simulink library "powerlib_models"  (Simulink 6.0)
settings: Solver=ode45  SolverMode=SingleTasking  StartTime=0.0  StopTime=10.0  RelTol=1e-3
values from neighbouring files (symbols this model uses):
  Ts = get(handles.edit1,'string')    [powergui.m]
undefined symbols (not defined in the file or in its folder): A, a0, a1, a2, a3, a4, a5, Ac, Amplitude, Amplitudes, B, BaseCurrent, BaseFlux, Bc, C, Capacitance, Cc, Columns, ConnectionType, Cs, ctrl, current, Current, damp, Dc, Dd, DiscIntNeverNeededParam, dref, dwo, exc, excAxis, F, Flux, fnom, Frequency, FreqVps, Gain1, gate, GH, GHd, GI, GId, GL, GLd, H, HarmonicGeneration, HT, hyd, I1_init, ib, ib2, Id1o, Inductance, InitialFlux, InitialSlope, io, Iq1o, isfinite, j, J ... (+138)
libraries: powerlib_models x32, powerlib_extras x4
(part 1 of 11)
settings Model: RequirementInfo=9  Creator=Patrice Brunelle  LastModifiedBy=batserve  ModifiedComment=-- Tue Aug 22 15:28:00 2000 -- Version 1.317  ModifiedHistory=Powerlib_models  ExtModeAutoUpdateStatusClock=off
settings OptimizationCC: BooleanDataType=off
settings DebuggingCC: SolverPrmCheckMsg=none
settings HardwareCC: TargetUnknown=on

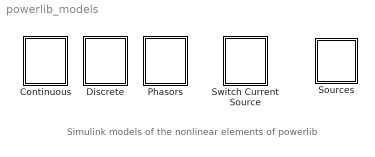
== system powerlib_models ==
  note: Simulink models of the nonlinear elements of powerlib
  Continuous : Subsystem
  Discrete : Subsystem
  Phasors : Subsystem
  Sources : Subsystem
  Switch Current Source : Subsystem

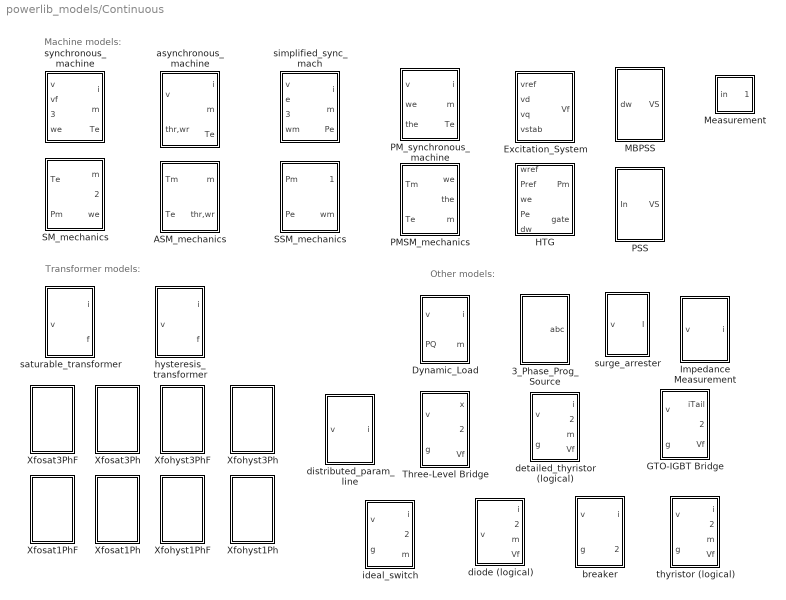
== system powerlib_models/Continuous ==
  note: Machine models:
  note: Transformer models:
  note: Other models:
  3_Phase_Prog_Source : Subsystem
  ASM_mechanics : Subsystem
  Dynamic_Load : Subsystem
  Excitation_System : Subsystem  mask(Excitation System){tr=tr, reg=reg, exc=exc, tgr=tgr, damp=damp, sat=sat, lim=lim, v0=v0}
      mask prompts: tr "Low-pass filter time constant Tr(s):"; reg "Regulator gain and time constant [ Ka()  Ta(s) ]:"; exc "Exciter  [ Ke()  Te(s) ]:"; tgr "Transient gain reduction [ Tb(s)  Tc(s) ]:"; damp "Damping filter gain and time constant  [ Kf()  Tf(s)  ]:"; sat "Field saturation parameters [ A, B ]:"; lim "Regulator output limits and gain [ Efmin, Efmax (p.u.), Kp() ]:"; v0 "Initial values of terminal voltage  and field voltage [ Vt0 (pu) Vf0(pu) ] :"
      mask help:
      | Implements an IEEE type 1 synchronous machine voltage regulator combined to an exciter. This block uses the dq components of terminal voltage (Synchronous Machine block, measurement ouputs 9 and 10).
      |
      | 1st input: desired stator terminal voltage (p.u.);
      | 2nd input: vd component of the terminal voltage (p.u.);
      | 3rd input: vq component of the terminal voltage (p.u.);
      | 4th input: stabilization voltage from user-supplied
      |                  power system stabilizer (p.u.);
      |
      | output: field voltage vfd to be applied to the
      |              Synchronous Machine block's 2nd input (p.u.).
      mask init:
      | ka=reg(1);ta=reg(2);ke=exc(1);te=exc(2);tb=tgr(1);tc=tgr(2);kf=damp(1);tf=damp(2);efmin=lim(1);efmax=lim(2);a=sat(1);b=sat(2);kp=lim(3);
      mask Help: web(psbhelp);
  GTO-IGBT Bridge : Subsystem  mask(GTO & IGBT Bridge Logic){nb_arm=3, Tf=1e-006, Tt=2e-006, Cs=Inf, VFs=[0 0], Rsw=1}
      mask prompts: nb_arm "Number of bridge arms (1,2 or 3)"; Tf "Curent 10% fall time Tf (s) :"; Tt "Current tail time Tt (s) :"; Cs "Snubber Capacitance Cs (F):"; VFs "Forward voltages [ Vf Vfd ]"; Rsw "Device resistances"
      mask help:
      | Generates the switch status ( 0 or 1) and the tail currents for a forced-commutated two- level bridge using GTO/Diode or IGBT/Diode pairs.
      | Specify  3 arms (6 switches) for 3 phase bridge, 2 arms for 4 switches, or 1 arm.
      | To turn-off the tail current, specify Tf=0 and Tt=0.
      mask init:
      | Vf=VFs(1);
      | Vfd=VFs(2);
      | nb_switch=nb_arm*2;
      | if nb_arm==1,
      |    Selec_Diode=[2 1];
      | elseif nb_arm==2,
      |    Selec_Diode=[2 1 4 3];
      | elseif nb_arm==3,
      |    Selec_Diode=[2 1 4 3 6 5];
      | end
  HTG : Subsystem  mask(Hydraulic Turbine and Governor){sm=sm, gate=gate, reg=reg, hyd=hyd, dref=dref, po=po}
      mask prompts: sm "Servo-motor [ Ka()  Ta(sec) ]:"; gate "Gate opening limits [ gmin,gmax(pu)    vgmin,vgmax(pu/s) ]:"; reg "Permanent droop and regulator  [ Rp() Kp() Ki() Kd() Td(s) ]:"; hyd "Hydraulic turbine [ beta()  Tw(sec) ]:"; dref "Droop reference (0=power error, 1=gate opening):"; po "Initial mechanical power (pu):"
      mask help:
      | Implements a hydraulic turbine combined to a PID governor system.
      |
      | 1st input: desired speed (p.u.);
      | 2nd input: desired electrical power (p.u.);
      | 3rd input: synchronous machine's actual speed (p.u., measurement output 13 of SM block);
      | 4th input: synchronous machine's actual electrical power (p.u., measurement output 14 of SM block);
      | 5th input: synchronous machine's actual speed deviation with respect to nominal (%, measurement output 15 of SM block);
      |
      | 1st output: mechanical power to be applied to the Synchronous Machine block's 1st input (p.u.);
      | 2nd output: gate opening (p.u.).
      mask init:
      | ka=sm(1);ta=sm(2);gmin=gate(1);gmax=gate(2);vgmin=gate(3);vgmax=gate(4);Rp=reg(1);kp=reg(2);ki=reg(3);kd=reg(4);td=reg(5);beta=hyd(1);tw=hyd(2);go=po*(gmax-gmin);
      mask Help: web(psbhelp);
  Impedance Measurement : Subsystem
      mask Type: Impedance Measurement model
      mask Description: Simulink model for the Impedance Measurement block. The model  injects a null current in the circuit.
  MBPSS : Subsystem  mask(MB-PSS ){OperationMode=Detailed settings, Kg=Kg, GL=GL, GI=GI, GH=GH, GLd=GLd, TcLF=TcLF, GId=GId, TcIF=TcIF, GHd=GHd, TcHF=TcHF, LIM=LIM, Plot_On=off, MagdB_On=off, FreqRange=logspace(-2,2,500)}
      mask prompts: OperationMode "Mode of operation:"; Kg "Global gain:"; GL "Low frequency band: [ FL(Hz), KL ]"; GI "Intermediate frequency band: [ FI(Hz), KI ]"; GH "High frequency band: [ FH(Hz), KH ]"; GLd "Low frequency gains: [ KL1, KL2, KL ]"; TcLF "Low frequency  time constants (s):"; GId "Intermediate frequency gains: [ KI1, KI2, KI ]"; TcIF "Intermediate frequency time constants (s):"; GHd "High frequency gains: [ KH1, KH2, KH ]"; TcHF "High frequency time constants (s):"; LIM "Signals Limits(VLmax,VImax,VHmax,VSmax)"; Plot_On "Plot frequency response"; MagdB_On "Magnitude in dB"; FreqRange "Frequency range (Hz):"
      mask help:
      | This block implements a Multi-band Power System Stabilizer (MB-PSS). Two operation modes are available: Detailed setting and simplified setting (IEEE Std 421.5).
      |
      | Input (dw): Synchronous machine speed deviation with respect to nominal (pu).
      | Output: stabilization voltage (pu).
      |
      | Note:
      | When "Detailed settings" is used, the low(L)-, intermediate(I)- and high(H)-frequency time constants must be given in the following order:
      | Tx1 to Tx12 followed by Kx11 and Kx17 (where x=L, I or H). Look under mask to see in which transfer functions these time constants are used.
      mask init:
      | Detailed=0;
      | if OperationMode==2,
      | Detailed=1;
      | Kg=1;
      | KL1=GLd(1);KL2=GLd(:,2);KL=GLd(3);
      | TL1=TcLF(1);TL2=TcLF(2);TL3=TcLF(3);TL4=TcLF(4);
      | TL5=TcLF(5);TL6=TcLF(6);TL7=TcLF(7);TL8=TcLF(8);
      | TL9=TcLF(9);TL10=TcLF(10);TL11=TcLF(11);TL12=TcLF(12);
      | KL11=TcLF(13);KL17=TcLF(14);
      | KI1=GId(1);KI2=GId(:,2);KI=GId(3);
      | TI1=TcIF(1);TI2=TcIF(2);TI3=TcIF(3);TI4=TcIF(4);
      | TI5=TcIF(5);TI6=TcIF(6);TI7=TcIF(7);TI8=TcIF(8);
      | TI9=TcIF(9);TI10=TcIF(10);TI11=TcIF(11);TI12=TcIF(12);
      | KI11=TcIF(13);KI17=TcIF(14);
      | KH1=GHd(1);KH2=GHd(:,2);KH=GHd(3);
      | TH1=TcHF(1);TH2=TcHF(2);TH3=TcHF(3);TH4=TcHF(4);
      | TH5=TcHF(5);TH6=TcHF(6);TH7=TcHF(7);TH8=TcHF(8);
      | TH9=TcHF(9);TH10=TcHF(10);TH11=TcHF(11);TH12=TcHF(12);
      | KH11=TcHF(13);KH17=TcHF(14);
      | else
      | %
      | R=1.2;K=(R*R+R)/(R*R-2*R+1);KL1=K;KL2=K;KI1=K;KI2=K;KH1=K;KH2=K;
      | TL2=1/(2*pi*GL(1)*sqrt(R));KL=GL(2);TL1=TL2/R;TL7=TL2;TL8=TL7*R;
      | %
      | TI2=1/(2*pi*GI(1)*sqrt(R));KI=GI(2);TI1=TI2/R;TI7=TI2;TI8=TI7*R;
      | TH2=1/(2*pi*GH(1)*sqrt(R));KH=GH(2);TH1=TH2/R;TH7=TH2;TH8=TH7*R;
      | %
      | TL3=0;TL4=0;TL5=0;TL6=0;TL9=0;TL10=0;TL11=0;TL12=0;
      | TI3=0;TI4=0;TI5=0;TI6=0;TI9=0;TI10=0;TI11=0;TI12=0;
      | TH3=0;TH4=0;TH5=0;TH6=0;TH9=0;TH10=0;TH11=0;TH12=0;
      | KL11=1;KL17=1;KI11=1;KI17=1;KH11=1;KH17=1;
      | end
      | LIM_VL=LIM(1);LIM_VI=LIM(2);LIM_VH=LIM(3);LIM_VS=LIM(4);
      | %
      | % LF Transfer function
      | numLF1=[TL1 KL11];
      | denLF1=[TL2 1];
      | sysLF1=tf(numLF1,denLF1);
      | numLF2=[TL3 1];
      | denLF2=[TL4 1];
      | sysLF2=tf(numLF2,denLF2);
      | numLF3=[TL5 1];
      | denLF3=[TL6 1];
      | sysLF3=tf(numLF3,denLF3);
      | numLF4=[TL7 KL17];
      | denLF4=[TL8 1];
      | sysLF4=tf(numLF4,denLF4);
      | numLF5=[TL9 1];
      | denLF5=[TL10 1];
      | sysLF5=tf(numLF5,denLF5);
      | numLF6=[TL11 1];
      | denLF6=[TL12 1];
      | sysLF6=tf(numLF6,denLF6);
      | %
      | sysLF=Kg*KL*((KL1*sysLF1*sysLF2*sysLF3) - (KL2*sysLF4*sysLF5*sysLF6));
      | %
      | %
      | % IF transfer function
      | numIF1=[TI1 KI11];
      | denIF1=[TI2 1];
      | sysIF1=tf(numIF1,denIF1);
      | numIF2=[TI3 1];
      | denIF2=[TI4 1];
      | sysIF2=tf(numIF2,denIF2);
      | numIF3=[TI5 1];
      | denIF3=[TI6 1];
      | sysIF3=tf(numIF3,denIF3);
      | numIF4=[TI7 KI17];
      | denIF4=[TI8 1];
      | sysIF4=tf(numIF4,denIF4);
      | numIF5=[TI9 1];
      | denIF5=[TI10 1];
      | sysIF5=tf(numIF5,denIF5);
      | numIF6=[TI11 1];
      | denIF6=[TI12 1];
      | sysIF6=tf(numIF6,denIF6);
      | %
      | sysIF=Kg*KI*((KI1*sysIF1*sysIF2*sysIF3) - (KI2*sysIF4*sysIF5*sysIF6));
      | %
      | %
      | % HF transfer function
      | numHF1=[TH1 KH11];
      | denHF1=[TH2 1];
      | sysHF1=tf(numHF1,denHF1);
      | numHF2=[TH3 1];
      | denHF2=[TH4 1];
      | sysHF2=tf(numHF2,denHF2);
      | numHF3=[TH5 1];
      | denHF3=[TH6 1];
      | sysHF3=tf(numHF3,denHF3);
      | numHF4=[TH7 KH17];
      | denHF4=[TH8 1];
      | sysHF4=tf(numHF4,denHF4);
      | numHF5=[TH9 1];
      | denHF5=[TH10 1];
      | sysHF5=tf(numHF5,denHF5);
      | numHF6=[TH11 1];
      | denHF6=[TH12 1];
      | sysHF6=tf(numHF6,denHF6);
      | %
      | sysHF=Kg*KH*((KH1*sysHF1*sysHF2*sysHF3) - (KH2*sysHF4*sysHF5*sysHF6));
      | %
      | %
      | % Input filter LIF
      | numLIFin=[1.759e-3 1];
      | denLIFin=[1.2739e-4 1.7823e-2 1];
      | sysLIFin=tf(numLIFin,denLIFin);
      | % Input filter HF
      | numHFin=[80 0 0];
      | denHFin=[1 82 161 80];
      | sysHFin=tf(numHFin,denHFin);
      | %
      | % Global transfer function:
      | sysL=sysLIFin*sysLF;
      | sysI=sysLIFin*sysIF;
      | sysH=sysHFin*sysHF;
      | sysG=sysL+sysI + sysH;
      | %
      | % Plot frequency response:
      | if Plot_On==1,
      |     w=2*pi*FreqRange;
      |     [MagL,PhaseL]=bode(sysL,w);
      |     [MagI,PhaseI]=bode(sysI,w);
      |     [MagH,PhaseH]=bode(sysH,w);
      |     [MagG,PhaseG]=bode(sysG,w);
      |     subplot(2,1,1)
      |      if  MagdB_On==1,
      |         YL= 20*log10(squeeze(MagL)) ;
      |         YI= 20*log10(squeeze(MagI)) ;
      |         YH= 20*log10(squeeze(MagH)) ;
      |         YG= 20*log10(squeeze(MagG)) ;
      |          strLabel='dB';
      | else
      | YL=squeeze(MagL);
      | YI=squeeze(MagI);
      | YH=squeeze(MagH);
      | YG=squeeze(MagG);
      | strLabel='pu/pu';
      | end
      | semilogx(FreqRange,YL,'m',FreqRange,YI,'g',FreqRange,YH,'b',FreqRange,YG,'r')
      | ylabel(strLabel);grid;
      | legend('LF band','IF band','HF band','Global',2);
      | title('PSS Frequency Response');
      |  subplot(2,1,2);
      | semilogx(FreqRange,rem(squeeze(PhaseL),360),'m',FreqRange,rem(squeeze(PhaseI),360),'g',FreqRange,rem(squeeze(PhaseH),360),'b',FreqRange,rem(squeeze(PhaseG),360),'r');
      | ylabel('Degrees');grid;
      | xlabel('Frequency (Hz)');
      | end
      mask StyleString: popup(Simplified settings|Detailed settings),edit,edit,edit,edit,edit,edit,edit,edit,edit,edit,edit,checkbox,checkbox,edit
      mask CallbackString: parametres=get_param(gcb,'MaskValues');p1=parametres{1};p13=parametres{13};if strcmp(p1,'Detailed settings');param2='off';param3='off';param4='off';param5='off';param6='on';param7='on';param8='on';param9='on';param10='on';param11='on';else;param2='on';param3='on';param4='on';param5='on';param6='off';param7='off';param8='off';param9='off';param10='off';param11='off';end;if strcmp(p13,'on');param14='on';param15='on';else;param14='off';param15='off';end;visible={'on',param2,param3,param4,param5,param6,param7,param8,param9,param10,param11,'on','on',param14,param15};set_param(gcb,'MaskVisibilities',visible)||||||||||||parametres=get_param(gcb,'MaskValues');p1=parametres{1};p13=parametres{13};if strcmp(p1,'Detailed settings');param2='off';param3='off';param4='off';param5='off';param6='on';param7='on';param8='on';param9='on';param10='on';param11='on';else;param2='on';param3='on';param4='on';param5='on';param6='off';param7='off';param8='off';param9='off';param10='off';param11='off';end;if strcmp(p13,'on');param14='on';param15='on';else;param14='off';param15='off';end;visible={'on',param2,param3,param4,param5,param6,param7,param8,param9,param10,param11,'on','on',param14,param15};set_param(gcb,'MaskVisibilities',visible)||
  Measurement : Subsystem
  PMSM_mechanics : Subsystem
  PM_synchronous_machine : Subsystem
  PSS : Subsystem  mask(Generic PSS){Tsensor=Tsensor, K=K, Twashout=Twashout, Tleadlag1=Tleadlag1, Tleadlag2=Tleadlag2, VSlimits=VSlimits, Vinit=Vinit, Plot_On=off, MagdB_On=on, FreqRange=logspace(-2,2,500)}
      mask prompts: Tsensor "Sensor time constant:"; K "Gain:"; Twashout "Wash-out time constant:"; Tleadlag1 "Lead-lag #1 time constants: [ Tnum Tden ]"; Tleadlag2 "Leag-lag #2 time constants: [ Tnum Tden ]"; VSlimits "Output limits: [ VSmin VSmax ]"; Vinit "Initial input:"; Plot_On "Plot frequency response"; MagdB_On "Magnitude in dB"; FreqRange "Frequency range (Hz):"
      mask help:
      | This block implements a generic Power System Stabilizer (PSS).
      |
      | Input (In): Synchronous machine speed deviation with respect to nominal (dw in pu) or acceleration power (Pa=Pm-Pe in pu).
      | Output (VS): stabilization voltage (pu).
      |
      | Look under mask to see how the various transfer functions are connected.
      mask init:
      | T1n=Tleadlag1(1);
      | T1d=Tleadlag1(2);
      | T2n=Tleadlag2(1);
      | T2d=Tleadlag2(2);
      | %
      | if Plot_On==1,
      | % Compute global system (sysG):
      | numS=[1];
      | denS=[Tsensor 1];
      | sysS=tf(numS,denS);
      | numW=[Twashout 0];
      | denW=[Twashout 1];
      | sysW=tf(numW,denW);
      | numL1=[T1n 1];
      | denL1=[T1d 1];
      | sysL1=tf(numL1,denL1);
      | numL2=[T2n 1];
      | denL2=[T2d 1];
      | sysL2=tf(numL2,denL2);
      | sysG=sysS*K*sysW*sysL1*sysL2;
      | %
      | % Plot response:
      | w=2*pi*FreqRange;
      | [Mag,Pha]=bode(sysG,w);
      | subplot(2,1,1)
      | if  MagdB_On==1,
      | Y= 20*log10(squeeze(Mag)) ;
      | strLabel='dB';
      | else
      | Y=squeeze(Mag);
      | strLabel='pu/pu';
      | end
      | %
      | semilogx(FreqRange,Y)
      | ylabel(strLabel);grid;
      | title('PSS Frequency Response');
      | subplot(2,1,2);
      | semilogx(FreqRange,rem(squeeze(Pha),360))
      | ylabel('Degrees');grid;
      | xlabel('Frequency (Hz)');
      | end
      mask CallbackString: |||||||parametres=get_param(gcb,'MaskValues');p8=parametres{8};if strcmp(p8,'on');param9='on';param10='on';else;param9='off';param10='off';end;visible={'on','on','on','on','on','on','on','on',param9,param10};set_param(gcb,'MaskVisibilities',visible)||
  SM_mechanics : Subsystem
  SSM_mechanics : Subsystem
  Three-Level Bridge : Subsystem  mask(Three-level Bridge Logic){nb_arm=nb_arm, Cs=Cs, Par_Vf=[Vf Vfd], Ron=Ron, Ts=0}
      mask prompts: nb_arm "Number of bridge arms (1,2 or 3)"; Cs "Snubber capacitance Cs (F):"; Par_Vf "Forward Voltages [ Vf  Vfd ]:"; Ron "Internal resistance Ron (Ohms):"; Ts "Sample time"
      mask init:
      | if nb_arm==1,
      |    StatusElements=[1 2 3];
      | elseif nb_arm==2,
      |    StatusElements=[1 2 5 3 4 6];
      | elseif nb_arm==3,
      |    StatusElements=[1 2 7 3 4 8 5 6 9];
      | end
  Xfohyst1Ph : Subsystem
      settings: CopyFcn=powericon('psbloadfunction',gcb,'NWindingsTransformerNoFlux','UpdateGotoTag');
  Xfohyst1PhF : Subsystem
      settings: CopyFcn=powericon('psbloadfunction',gcb,'NWindingsTransformerFlux','UpdateGotoTag');
  Xfohyst3Ph : Subsystem
      settings: CopyFcn=powericon('psbloadfunction',gcb,'ThreePhaseTransformerNoFlux','UpdateGotoTag');
  Xfohyst3PhF : Subsystem
      settings: CopyFcn=powericon('psbloadfunction',gcb,'ThreePhaseTransformerFlux','UpdateGotoTag');
  Xfosat1Ph : Subsystem
      settings: CopyFcn=powericon('psbloadfunction',gcb,'NWindingsTransformerNoFlux','UpdateGotoTag');
  Xfosat1PhF : Subsystem
      settings: CopyFcn=powericon('psbloadfunction',gcb,'NWindingsTransformerFlux','UpdateGotoTag');
  Xfosat3Ph : Subsystem
      settings: CopyFcn=powericon('psbloadfunction',gcb,'ThreePhaseTransformerNoFlux','UpdateGotoTag');
  Xfosat3PhF : Subsystem
      settings: CopyFcn=powericon('psbloadfunction',gcb,'ThreePhaseTransformerFlux','UpdateGotoTag');
  asynchronous_machine : Subsystem
  breaker : Subsystem  mask{Nsw=1, istate=0, Rsw=1}
      mask prompts: Nsw "Number of breakers"; istate "Initial state"; Rsw "Breaker Resistances"
      mask help: Simulink model for the Breaker block
  detailed_thyristor (logical) : Subsystem  mask{Nsw=1, Vf=0, Rsw=1}
      mask prompts: Nsw "Number of thyristors"; Vf "Forward voltage Vf (V)"; Rsw "Thyristor resistances"
      mask help: Simulink model for the Detailed Thyristor block when Lon=0. This model is used during a continuous simulation.
  diode (logical) : Subsystem  mask{Nsw=1, Vf=0, Rsw=1}
      mask prompts: Nsw "Number of Diodes"; Vf "Forward voltage Vf (V):"; Rsw "Diode resistances"
      mask help: Simulink model for the Diode block when Lon=0. This model is used during a continuous simulation.
  distributed_param_line : Subsystem  mask(Distributed Parameter Line Model){nphase=Phases, f=Frequency, ri=Resistance, li=Inductance, ci=Capacitance, long=Length, V1_init=x1, V2_init=x2, I1_init=x3, I2_init=x4, time_init=x5}
      mask prompts: nphase "Number of phases"; f "Frequency used for R L C specification (Hz)"; ri "R [3*3 matrix] or [R0 R1] (ohms/km)"; li "L [3*3matrix ] or [L0 L1] (H/km)"; ci "C [3*3matrix] or [C0 C1] (F/km)"; long "Line length (km)"; time_init "time delay init"
      mask help: Simulink model for the Distributed Parameter Line block. The last five parameters are automatically calculated by SimPowerSystems at the begining of the simulation.
      mask init:
      | [Zm,R,v,Ti]=powericon('Distributed Parameter Line Model',nphase,f,ri,li,ci);to=long./v;Rt4=R*long/4;h=(Zm-Rt4)./(Zm+Rt4);
  hysteresis_transformer : Subsystem  mask{SaturationFlux=SaturationFlux, SaturationCurrent=SaturationCurrent, InitialFlux=InitialFlux, FluxBase=BaseFlux, CurrentBase=BaseCurrent, Tolerances=Tolerances, HT=HT, UpperFlux=UpperFlux, LowerFlux=LowerFlux, Current=Current, InitialSlope=InitialSlope, TransfoNumber=TransfoNumber, sfun_InitialFlux=sfun_InitialFlux}
      mask prompts: SaturationFlux "Saturation Flux"; SaturationCurrent "Saturation Current"; InitialFlux "Initial Flux"; InitialSlope "Initial Slope"; TransfoNumber "Transfo Number"
  ideal_switch : Subsystem  mask(Switch logic model){Nsw=1, Rsw=1}
      mask prompts: Nsw "Number of switches"; Rsw "Switch resistances"
      mask help: Simulink model for the Ideal Switch block during a continuous simulation. The switching logic of the ideal switch is handled by the sfun_psbcontc.c function.
  saturable_transformer : Subsystem  mask{SaturationFlux=SaturationFlux, SaturationCurrent=SaturationCurrent, InitialFlux=InitialFlux}
      mask prompts: SaturationFlux "Saturation Flux"; SaturationCurrent "Saturation Current"; InitialFlux "Initial Flux"
  simplified_sync_mach : Subsystem
  surge_arrester : Subsystem  mask(Surge arrester model){uref=ProtectionVoltage, n=Columns, iref=ReferenceCurrent, param1=Segment1, param2=Segment2, param3=Segment3, BreakLoop=1}
      mask prompts: uref "Protection voltage  (V):"; n "Number of columns:"; iref "Nominal current per column  (A):"; param1 "Segment 1 characteristics: [ k1 alpha1 ]"; param2 "Segment 2 characteristics: [ k2 alpha2 ]"; param3 "Segment 3 characteristics: [ k3 alpha3 ]"; BreakLoop "Break algebraic loop:"
      mask help: Simulink model for the Surge Arrester block (Metal oxide varistor).
      mask init:
      | k1=param1(1);
      | k2=param2(1);
      | k3=param3(1);
      | a1=round(param1(2));
      | a2=round(param2(2));
      | a3=round(param3(2));
      | p1=iref*n/(k1^a1);
      | p2=iref*n/(k2^a2);
      | p3=iref*n/(k3^a3);
      | ic1=p1*((p1/p2)^(a1/(a2-a1)));
      | ic2=p2*((p2/p3)^(a2/(a3-a2)));
      | % Break Alg. Loop:
  synchronous_machine : Subsystem
  thyristor (logical) : Subsystem  mask{Nsw=1, Vf=0, Rsw=1}
      mask prompts: Nsw "Number of thyristors"; Vf "Forward Voltage Vf(V):"; Rsw "Thyristor resistances"
      mask help: Simulink model for the Thyristor block when Lon=0. This model is used during a continuous simulation.

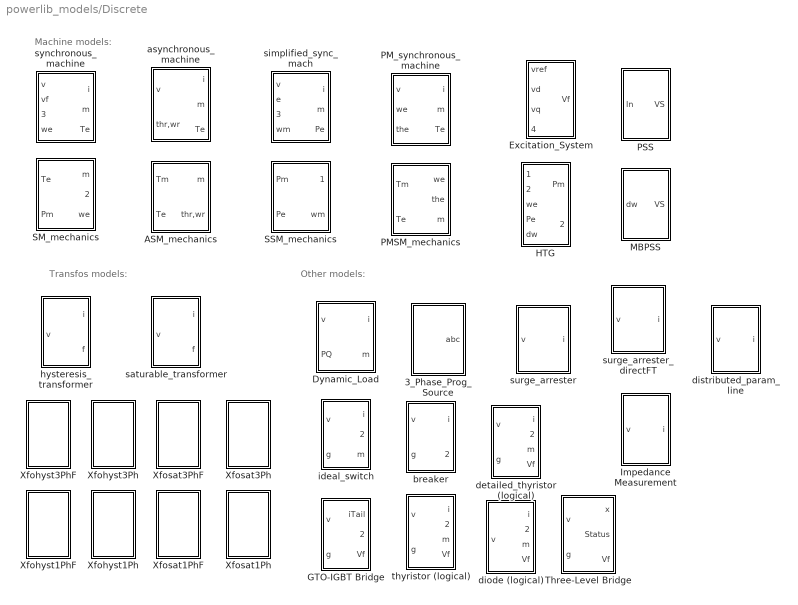
== system powerlib_models/Discrete ==
  note: Machine models:
  note: Transfos models:
  note: Other models:
  3_Phase_Prog_Source : Subsystem
  ASM_mechanics : Subsystem
  Dynamic_Load : Subsystem
  Excitation_System : Subsystem  mask(Discrete Excitation System){tr=tr, reg=reg, exc=exc, tgr=tgr, damp=damp, sat=sat, lim=lim, v0=v0, Ts=50e-6}
      mask prompts: tr "Low-pass filter time constant Tr(s):"; reg "Regulator gain and time constant [ Ka()  Ta(s) ]:"; exc "Exciter  [ Ke()  Te(s) ]:"; tgr "Transient gain reduction [ Tb(s)  Tc(s) ]:"; damp "Damping filter gain and time constant  [ Kf()  Tf(s)  ]:"; sat "Field saturation parameters [ A, B ]:"; lim "Regulator output limits and gain [ Efmin, Efmax (p.u.), Kp() ]:"; v0 "Initial values of terminal voltage  and field voltage [ Vt0 (pu) Vf0(pu) ] :"; Ts "Sample time:"
      mask help:
      | Implements an discrete IEEE type 1 synchronous machine voltage regulator combined to an exciter. This block uses the dq components of terminal voltage (Synchronous Machine block, measurement ouputs 9 and 10).
      |
      | 1st input: desired stator terminal voltage (p.u.);
      | 2nd input: vd component of the terminal voltage (p.u.);
      | 3rd input: vq component of the terminal voltage (p.u.);
      | 4th input: stabilization voltage from user-supplied
      |                  power system stabilizer (p.u.);
      |
      | output: field voltage vfd to be applied to the
      |              Synchronous Machine block's 2nd input (p.u.).
      mask init:
      | ka=reg(1);ta=reg(2);ke=exc(1);te=exc(2);tb=tgr(1);tc=tgr(2);kf=damp(1);tf=damp(2);efmin=lim(1);efmax=lim(2);a=sat(1);b=sat(2);kp=lim(3);
      | if te==0,
      | te=1e-6;
      | end
      mask Help: web(psbhelp);
  GTO-IGBT Bridge : Subsystem  mask(GTO & IGBT Bridge Logic){nb_arm=3, Tf=0, Tt=0, Cs=Inf, VFs=[0 0], Rsw=1, Ts=1}
      mask prompts: nb_arm "Number of bridge arms (1,2 or 3)"; Tf "Curent 10% fall time Tf (s) :"; Tt "Current tail time Tt (s) :"; Cs "Snubber Capacitance Cs (F):"; VFs "Forward Voltages [ Vf  Vfd ]"; Rsw "Device resistance"; Ts "Time step Ts (s) :"
      mask help:
      | Generates the switch status ( 0 or 1) and the tail currents for a forced-commutated two- level bridge using GTO/Diode or IGBT/Diode pairs.
      | Specify  3 arms (6 switches) for 3 phase bridge, 2 arms for 4 switches, or 1 arm.
      | To turn-off the tail current, specify Tf=0 and Tt=0.
      mask init:
      | Vf=VFs(1);
      | Vfd=VFs(2);
      | nb_switch=nb_arm*2;
      | if nb_arm==1,
      |    Selec_Diode=[2 1];
      | elseif nb_arm==2,
      |    Selec_Diode=[2 1 4 3];
      | elseif nb_arm==3,
      |    Selec_Diode=[2 1 4 3 6 5];
      | end
  HTG : Subsystem  mask(Discrete Hydraulic Turbine and Governor){sm=sm, gate=gate, reg=reg, hyd=hyd, dref=dref, po=po, Ts=50e-6}
      mask prompts: sm "Servo-motor [ Ka()  Ta(sec) ]:"; gate "Gate opening limits [ gmin,gmax(pu)    vgmin,vgmax(pu/s) ]:"; reg "Permanent droop and regulator  [ Rp() Kp() Ki() Kd() Td(s) ]:"; hyd "Hydraulic turbine [ beta()  Tw(sec) ]:"; dref "Droop reference (0=power error, 1=gate opening):"; po "Initial mechanical power (pu):"; Ts "Sample time:"
      mask help:
      | Implements a discrete hydraulic turbine combined to a discrete PID governor system.
      |
      | 1st input: desired speed (p.u.);
      | 2nd input: desired electrical power (p.u.);
      | 3rd input: synchronous machine's actual speed (p.u., measurement output 13 of SM block);
      | 4th input: synchronous machine's actual electrical power (p.u., measurement output 14 of SM block);
      | 5th input: synchronous machine's actual speed deviation with respect to nominal (%, measurement output 15 of SM block);
      |
      | 1st output: mechanical power to be applied to the Synchronous Machine block's 1st input (p.u.);
      | 2nd output: gate opening (p.u.).
      mask init:
      | ka=sm(1);ta=sm(2);gmin=gate(1);gmax=gate(2);vgmin=gate(3);vgmax=gate(4);Rp=reg(1);kp=reg(2);ki=reg(3);kd=reg(4);td=reg(5);beta=hyd(1);tw=hyd(2);go=po*(gmax-gmin);
      mask Help: web(psbhelp);
  Impedance Measurement : Subsystem
      mask Type: Impedance Measurement model
      mask Description: The impedance Measurement block injects a null current in the circuit.
  MBPSS : Subsystem  mask(MB-PSS ){OperationMode=Detailed settings, Kg=Kg, GL=GL, GI=GI, GH=GH, GLd=GLd, TcLF=TcLF, GId=GId, TcIF=TcIF, GHd=GHd, TcHF=TcHF, LIM=LIM, Plot_On=off, MagdB_On=off, FreqRange=logspace(-2,2,500), Ts=50e-6}
      mask prompts: OperationMode "Mode of operation:"; Kg "Global gain:"; GL "Low frequency band: [ FL(Hz), KL ]"; GI "Intermediate frequency band: [ FI(Hz), KI ]"; GH "High frequency band: [ FH(Hz), KH ]"; GLd "Low frequency gains: [ KL1, KL2, KL ]"; TcLF "Low frequency  time constants (s):"; GId "Intermediate frequency gains: [ KI1, KI2, KI ]"; TcIF "Intermediate frequency time constants (s):"; GHd "High frequency gains: [ KH1, KH2, KH ]"; TcHF "High frequency time constants (s):"; LIM "Signals Limits(VLmax,VImax,VHmax,VSmax)"; Plot_On "Plot frequency response"; MagdB_On "Magnitude in dB"; FreqRange "Frequency range (Hz):"
      mask help:
      | This block implements a Multi-band Power System Stabilizer (MB-PSS). Two operation modes are available: Detailed setting and simplified setting (IEEE Std 421.5).
      |
      | Input (dw): Synchronous machine speed deviation with respect to nominal (pu).
      | Output: stabilization voltage (pu).
      |
      | Note:
      | When "Detailed settings" is used, the low(L)-, intermediate(I)- and high(H)-frequency time constants must be given in the following order:
      | Tx1 to Tx12 followed by Kx11 and Kx17 (where x=L, I or H). Look under mask to see in which transfer functions these time constants are used.
      mask init:
      | Detailed=0;
      | if OperationMode==2,
      | Detailed=1;
      | Kg=1;
      | KL1=GLd(1);KL2=GLd(:,2);KL=GLd(3);
      | TL1=TcLF(1);TL2=TcLF(2);TL3=TcLF(3);TL4=TcLF(4);
      | TL5=TcLF(5);TL6=TcLF(6);TL7=TcLF(7);TL8=TcLF(8);
      | TL9=TcLF(9);TL10=TcLF(10);TL11=TcLF(11);TL12=TcLF(12);
      | KL11=TcLF(13);KL17=TcLF(14);
      | KI1=GId(1);KI2=GId(:,2);KI=GId(3);
      | TI1=TcIF(1);TI2=TcIF(2);TI3=TcIF(3);TI4=TcIF(4);
      | TI5=TcIF(5);TI6=TcIF(6);TI7=TcIF(7);TI8=TcIF(8);
      | TI9=TcIF(9);TI10=TcIF(10);TI11=TcIF(11);TI12=TcIF(12);
      | KI11=TcIF(13);KI17=TcIF(14);
      | KH1=GHd(1);KH2=GHd(:,2);KH=GHd(3);
      | TH1=TcHF(1);TH2=TcHF(2);TH3=TcHF(3);TH4=TcHF(4);
      | TH5=TcHF(5);TH6=TcHF(6);TH7=TcHF(7);TH8=TcHF(8);
      | TH9=TcHF(9);TH10=TcHF(10);TH11=TcHF(11);TH12=TcHF(12);
      | KH11=TcHF(13);KH17=TcHF(14);
      | else
      | %
      | R=1.2;K=(R*R+R)/(R*R-2*R+1);KL1=K;KL2=K;KI1=K;KI2=K;KH1=K;KH2=K;
      | TL2=1/(2*pi*GL(1)*sqrt(R));KL=GL(2);TL1=TL2/R;TL7=TL2;TL8=TL7*R;
      | %
      | TI2=1/(2*pi*GI(1)*sqrt(R));KI=GI(2);TI1=TI2/R;TI7=TI2;TI8=TI7*R;
      | TH2=1/(2*pi*GH(1)*sqrt(R));KH=GH(2);TH1=TH2/R;TH7=TH2;TH8=TH7*R;
      | %
      | TL3=0;TL4=0;TL5=0;TL6=0;TL9=0;TL10=0;TL11=0;TL12=0;
      | TI3=0;TI4=0;TI5=0;TI6=0;TI9=0;TI10=0;TI11=0;TI12=0;
      | TH3=0;TH4=0;TH5=0;TH6=0;TH9=0;TH10=0;TH11=0;TH12=0;
      | KL11=1;KL17=1;KI11=1;KI17=1;KH11=1;KH17=1;
      | end
      | LIM_VL=LIM(1);LIM_VI=LIM(2);LIM_VH=LIM(3);LIM_VS=LIM(4);
      | %
      | % LF Transfer function
      | numLF1=[TL1 KL11];
      | denLF1=[TL2 1];
      | sysLF1=tf(numLF1,denLF1);
      | numLF2=[TL3 1];
      | denLF2=[TL4 1];
      | sysLF2=tf(numLF2,denLF2);
      | numLF3=[TL5 1];
      | denLF3=[TL6 1];
      | sysLF3=tf(numLF3,denLF3);
      | numLF4=[TL7 KL17];
      | denLF4=[TL8 1];
      | sysLF4=tf(numLF4,denLF4);
      | numLF5=[TL9 1];
      | denLF5=[TL10 1];
      | sysLF5=tf(numLF5,denLF5);
      | numLF6=[TL11 1];
      | denLF6=[TL12 1];
      | sysLF6=tf(numLF6,denLF6);
      | %
      | sysLF=Kg*KL*((KL1*sysLF1*sysLF2*sysLF3) - (KL2*sysLF4*sysLF5*sysLF6));
      | %
      | %
      | % IF transfer function
      | numIF1=[TI1 KI11];
      | denIF1=[TI2 1];
      | sysIF1=tf(numIF1,denIF1);
      | numIF2=[TI3 1];
      | denIF2=[TI4 1];
      | sysIF2=tf(numIF2,denIF2);
      | numIF3=[TI5 1];
      | denIF3=[TI6 1];
      | sysIF3=tf(numIF3,denIF3);
      | numIF4=[TI7 KI17];
      | denIF4=[TI8 1];
      | sysIF4=tf(numIF4,denIF4);
      | numIF5=[TI9 1];
      | denIF5=[TI10 1];
      | sysIF5=tf(numIF5,denIF5);
      | numIF6=[TI11 1];
      | denIF6=[TI12 1];
      | sysIF6=tf(numIF6,denIF6);
      | %
      | sysIF=Kg*KI*((KI1*sysIF1*sysIF2*sysIF3) - (KI2*sysIF4*sysIF5*sysIF6));
      | %
      | %
      | % HF transfer function
      | numHF1=[TH1 KH11];
      | denHF1=[TH2 1];
      | sysHF1=tf(numHF1,denHF1);
      | numHF2=[TH3 1];
      | denHF2=[TH4 1];
      | sysHF2=tf(numHF2,denHF2);
      | numHF3=[TH5 1];
      | denHF3=[TH6 1];
      | sysHF3=tf(numHF3,denHF3);
      | numHF4=[TH7 KH17];
      | denHF4=[TH8 1];
      | sysHF4=tf(numHF4,denHF4);
      | numHF5=[TH9 1];
      | denHF5=[TH10 1];
      | sysHF5=tf(numHF5,denHF5);
      | numHF6=[TH11 1];
      | denHF6=[TH12 1];
      | sysHF6=tf(numHF6,denHF6);
      | %
      | sysHF=Kg*KH*((KH1*sysHF1*sysHF2*sysHF3) - (KH2*sysHF4*sysHF5*sysHF6));
      | %
      | %
      | % Input filter LIF
      | numLIFin=[1.759e-3 1];
      | denLIFin=[1.2739e-4 1.7823e-2 1];
      | sysLIFin=tf(numLIFin,denLIFin);
      | % Input filter HF
      | numHFin=[80 0 0];
      | denHFin=[1 82 161 80];
      | sysHFin=tf(numHFin,denHFin);
      | %
      | % Global transfer function:
      | sysL=sysLIFin*sysLF;
      | sysI=sysLIFin*sysIF;
      | sysH=sysHFin*sysHF;
      | sysG=sysL+sysI + sysH;
      | %
      | % Plot frequency response:
      | if Plot_On==1,
      |     w=2*pi*FreqRange;
      |     [MagL,PhaseL]=bode(sysL,w);
      |     [MagI,PhaseI]=bode(sysI,w);
      |     [MagH,PhaseH]=bode(sysH,w);
      |     [MagG,PhaseG]=bode(sysG,w);
      |     subplot(2,1,1)
      |      if  MagdB_On==1,
      |         YL= 20*log10(squeeze(MagL)) ;
      |         YI= 20*log10(squeeze(MagI)) ;
      |         YH= 20*log10(squeeze(MagH)) ;
      |         YG= 20*log10(squeeze(MagG)) ;
      |          strLabel='dB';
      | else
      | YL=squeeze(MagL);
      | YI=squeeze(MagI);
      | YH=squeeze(MagH);
      | YG=squeeze(MagG);
      | strLabel='pu/pu';
      | end
      | semilogx(FreqRange,YL,'m',FreqRange,YI,'g',FreqRange,YH,'b',FreqRange,YG,'r')
      | ylabel(strLabel);grid;
      | legend('LF band','IF band','HF band','Global',2);
      | title('MB-PSS Frequency Response');
      |  subplot(2,1,2);
      | semilogx(FreqRange,rem(squeeze(PhaseL),360),'m',FreqRange,rem(squeeze(PhaseI),360),'g',FreqRange,rem(squeeze(PhaseH),360),'b',FreqRange,rem(squeeze(PhaseG),360),'r');
      | ylabel('Degrees');grid;
      | xlabel('Frequency (Hz)');
      | end
      mask StyleString: popup(Simplified settings|Detailed settings),edit,edit,edit,edit,edit,edit,edit,edit,edit,edit,edit,checkbox,checkbox,edit,edit
      mask CallbackString: parametres=get_param(gcb,'MaskValues');p1=parametres{1};p13=parametres{13};if strcmp(p1,'Detailed settings');param2='off';param3='off';param4='off';param5='off';param6='on';param7='on';param8='on';param9='on';param10='on';param11='on';else;param2='on';param3='on';param4='on';param5='on';param6='off';param7='off';param8='off';param9='off';param10='off';param11='off';end;if strcmp(p13,'on');param14='on';param15='on';else;param14='off';param15='off';end;visible={'on',param2,param3,param4,param5,param6,param7,param8,param9,param10,param11,'on','on',param14,param15,'on'};set_param(gcb,'MaskVisibilities',visible)||||||||||||parametres=get_param(gcb,'MaskValues');p1=parametres{1};p13=parametres{13};if strcmp(p1,'Detailed settings');param2='off';param3='off';param4='off';param5='off';param6='on';param7='on';param8='on';param9='on';param10='on';param11='on';else;param2='on';param3='on';param4='on';param5='on';param6='off';param7='off';param8='off';param9='off';param10='off';param11='off';end;if strcmp(p13,'on');param14='on';param15='on';else;param14='off';param15='off';end;visible={'on',param2,param3,param4,param5,param6,param7,param8,param9,param10,param11,'on','on',param14,param15,'on'};set_param(gcb,'MaskVisibilities',visible)|||
  PMSM_mechanics : Subsystem
  PM_synchronous_machine : Subsystem
  PSS : Subsystem  mask(Generic PSS){Tsensor=Tsensor, K=K, Twashout=Twashout, Tleadlag1=Tleadlag1, Tleadlag2=Tleadlag2, VSlimits=VSlimits, Vinit=Vinit, Plot_On=off, MagdB_On=on, FreqRange=logspace(-2,2,500), Ts=50e-6}
      mask prompts: Tsensor "Sensor time constant:"; K "Gain:"; Twashout "Wash-out time constant:"; Tleadlag1 "Lead-lag #1 time constants: [ Tnum Tden ]"; Tleadlag2 "Leag-lag #2 time constants: [ Tnum Tden ]"; VSlimits "Output limits: [ VSmin VSmax ]"; Vinit "Initial input:"; Plot_On "Plot frequency response"; MagdB_On "Magnitude in dB"; FreqRange "Frequency range (Hz):"
      mask help:
      | This block implements a generic Power System Stabilizer (PSS).
      |
      | Input (In): Synchronous machine speed deviation with respect to nominal (dw in pu) or acceleration power (Pa=Pm-Pe in pu).
      | Output (VS): stabilization voltage (pu).
      |
      | Look under mask to see how the various transfer functions are connected.
      mask init:
      | T1n=Tleadlag1(1);
      | T1d=Tleadlag1(2);
      | T2n=Tleadlag2(1);
      | T2d=Tleadlag2(2);
      | %
      | if Plot_On==1,
      | % Compute global system (sysG):
      | numS=[1];
      | denS=[Tsensor 1];
      | sysS=tf(numS,denS);
      | numW=[Twashout 0];
      | denW=[Twashout 1];
      | sysW=tf(numW,denW);
      | numL1=[T1n 1];
      | denL1=[T1d 1];
      | sysL1=tf(numL1,denL1);
      | numL2=[T2n 1];
      | denL2=[T2d 1];
      | sysL2=tf(numL2,denL2);
      | sysG=sysS*K*sysW*sysL1*sysL2;
      | %
      | % Plot response:
      | w=2*pi*FreqRange;
      | [Mag,Pha]=bode(sysG,w);
      | subplot(2,1,1)
      | if  MagdB_On==1,
      | Y= 20*log10(squeeze(Mag)) ;
      | strLabel='dB';
      | else
      | Y=squeeze(Mag);
      | strLabel='pu/pu';
      | end
      | %
      | semilogx(FreqRange,Y)
      | ylabel(strLabel);grid;
      | title('PSS Frequency Response');
      | subplot(2,1,2);
      | semilogx(FreqRange,rem(squeeze(Pha),360))
      | ylabel('Degrees');grid;
      | xlabel('Frequency (Hz)');
      | end
      mask CallbackString: |||||||parametres=get_param(gcb,'MaskValues');p8=parametres{8};if strcmp(p8,'on');param9='on';param10='on';else;param9='off';param10='off';end;visible={'on','on','on','on','on','on','on','on',param9,param10,'on'};set_param(gcb,'MaskVisibilities',visible)|||
  SM_mechanics : Subsystem
  SSM_mechanics : Subsystem
  Three-Level Bridge : Subsystem  mask(Three-level Bridge Logic){nb_arm=1, Cs=inf, Par_Vf=[0 0], Ron=1, Ts=1}
      mask prompts: nb_arm "Number of bridge arms (1,2 or 3)"; Cs "Snubber capacitance Cs (F):"; Par_Vf "Forward Voltages [ Vf  Vfd ]:"; Ron "Internal resistance Ron (Ohms):"; Ts "Sample time"
      mask init:
      | if nb_arm==1,
      |    StatusElements=[1 2 3];
      | elseif nb_arm==2,
      |    StatusElements=[1 2 5 3 4 6];
      | elseif nb_arm==3,
      |    StatusElements=[1 2 7 3 4 8 5 6 9];
      | end
  Xfohyst1Ph : Subsystem
      settings: CopyFcn=powericon('psbloadfunction',gcb,'NWindingsTransformerNoFlux','UpdateGotoTag');
  Xfohyst1PhF : Subsystem
      settings: CopyFcn=powericon('psbloadfunction',gcb,'NWindingsTransformerFlux','UpdateGotoTag');
  Xfohyst3Ph : Subsystem
      settings: CopyFcn=powericon('psbloadfunction',gcb,'ThreePhaseTransformerNoFlux','UpdateGotoTag');
  Xfohyst3PhF : Subsystem
      settings: CopyFcn=powericon('psbloadfunction',gcb,'ThreePhaseTransformerFlux','UpdateGotoTag');
  Xfosat1Ph : Subsystem
      settings: CopyFcn=powericon('psbloadfunction',gcb,'NWindingsTransformerNoFlux','UpdateGotoTag');
  Xfosat1PhF : Subsystem
      settings: CopyFcn=powericon('psbloadfunction',gcb,'NWindingsTransformerFlux','UpdateGotoTag');
  Xfosat3Ph : Subsystem
      settings: CopyFcn=powericon('psbloadfunction',gcb,'ThreePhaseTransformerNoFlux','UpdateGotoTag');
  Xfosat3PhF : Subsystem
      settings: CopyFcn=powericon('psbloadfunction',gcb,'ThreePhaseTransformerFlux','UpdateGotoTag');
  asynchronous_machine : Subsystem
  breaker : Subsystem  mask(Breaker Model){Nsw=1, istate=0, Rsw=1, Ts=1}
      mask prompts: Nsw "Number of breaker"; istate "Initial state"; Rsw "Breaker resistances"; Ts "Sample time (s):"
      mask help: Simulink model for the Breaker block.
  detailed_thyristor (logical) : Subsystem  mask(thyristors logic model){Nsw=1, Vf=0, Rsw=1, Ts=1}
      mask prompts: Nsw "Number of thyristors"; Vf "Forward voltage Vf (V):"; Rsw "Thyristor resistances"; Ts "Sample time (s):"
  diode (logical) : Subsystem  mask(Diode logic model){Nsw=1, Vf=0, Rsw=1, Ts=1}
      mask prompts: Nsw "Number of diodes"; Vf "Forward Voltage Vf (V):"; Rsw "Diode resistances"; Ts "Sample time (s):"
  distributed_param_line : Subsystem  mask(Distributed Parameter Line Model){nphase=Phases, f=Frequency, ri=Resistance, li=Inductance, ci=Capacitance, long=Length, V1_init=x1, V2_init=x2, I1_init=x3, I2_init=x4, time_init=x5}
      mask prompts: nphase "Number of phases"; f "Frequency used for R L C specification (Hz)"; ri "R [3*3 matrix] or [R0 R1] (ohms/km)"; li "L [3*3matrix ] or [L0 L1] (H/km)"; ci "C [3*3matrix] or [C0 C1] (F/km)"; long "Line length (km)"; time_init "time delay init"
      mask help: N phases distributed parameters line with losses
      mask init:
      | [Zm,R,v,Ti]=powericon('Distributed Parameter Line Model',nphase,f,ri,li,ci);to=long./v;Rt4=R*long/4;h=(Zm-Rt4)./(Zm+Rt4);
      mask Help:
      | Multiphase distributed parameter line.  For symetrical or asymetrical lines, R L and C parameters are specified by NxN matrices
      | For 2-phase, 3-phase and six-phase symetrical lines, R L C parameters can be also specified by sequence component vectors:  ie [R0 R1] for 2 and 3 phase line or [R1 R0 R0m] for a six-phase line representing two identical coupled 3-phase circuits.
  hysteresis_transformer : Subsystem  mask{SaturationFlux=SaturationFlux, SaturationCurrent=SaturationCurrent, InitialFlux=InitialFlux, FluxBase=BaseFlux, CurrentBase=BaseCurrent, Tolerances=Tolerances, HT=HT, UpperFlux=UpperFlux, LowerFlux=LowerFlux, Current=Current, InitialSlope=InitialSlope, TransfoNumber=TransfoNumber, Ts=Ts, sfun_InitialFlux=sfun_InitialFlux}
      mask prompts: InitialFlux "Initial Flux"; TransfoNumber "Transfo Number"
  ideal_switch : Subsystem  mask(Switch logic model){Nsw=1, Rsw=1, Ts=1}
      mask prompts: Nsw "Number of Ideal Switches"; Rsw "Switchr resistances"; Ts "Sample Time (s)"
  saturable_transformer : Subsystem  mask{SaturationFlux=SaturationFlux, SaturationCurrent=SaturationCurrent, InitialFlux=InitialFlux, Ts=Ts}
      mask prompts: SaturationFlux "Saturation Flux"; SaturationCurrent "Saturation Current"; InitialFlux "Initial Flux"
  simplified_sync_mach : Subsystem
  surge_arrester : Subsystem  mask(Surge arrester model){uref=ProtectionVoltage, n=Columns, iref=ReferenceCurrent, param1=Segment1, param2=Segment2, param3=Segment3, Ts=Ts}
      mask prompts: uref "Protection voltage  (V):"; n "Number of columns:"; iref "Nominal current per column  (A):"; param1 "Segment 1 characteristics: [ k1 alpha1 ]"; param2 "Segment 2 characteristics: [ k2 alpha2 ]"; param3 "Segment 3 characteristics: [ k3 alpha3 ]"; Ts "Sample Time (s)"
      mask help: The surge arrester model is a Metal oxide varistor.
      mask init:
      | k1=param1(1);k2=param2(1);k3=param3(1);a1=round(param1(2));a2=round(param2(2));a3=round(param3(2));p1=iref*n/(k1^a1); p2=iref*n/(k2^a2); p3=iref*n/(k3^a3); ic1=p1*((p1/p2)^(a1/(a2-a1)));ic2=p2*((p2/p3)^(a2/(a3-a2)));
  surge_arrester_directFT : Subsystem  mask(Surge arrester model){uref=ProtectionVoltage, n=Columns, iref=ReferenceCurrent, param1=Segment1, param2=Segment2, param3=Segment3, Ts=Ts}
      mask prompts: uref "Protection voltage  (V):"; n "Number of columns:"; iref "Nominal current per column  (A):"; param1 "Segment 1 characteristics: [ k1 alpha1 ]"; param2 "Segment 2 characteristics: [ k2 alpha2 ]"; param3 "Segment 3 characteristics: [ k3 alpha3 ]"; Ts "Sample Time (s)"
      mask help: The surge arrester model is a Metal oxide varistor.
      mask init: same as powerlib_models/Discrete/surge_arrester
  synchronous_machine : Subsystem
  thyristor (logical) : Subsystem  mask(thyristors logic model){Nsw=1, Vf=0, Rsw=1, Ts=1}
      mask prompts: Nsw "Number of thyristors"; Vf "Forward voltage Vf (V)"; Rsw "Thyristor resistances"; Ts "Sample time (s):"

== system powerlib_models/Phasors ==
  note: Machine models:
  3_Phase_Prog_Source : Subsystem
  ASM_mechanics : Subsystem
  Dynamic_Load : Subsystem
  Impedance Measurement : Subsystem
      mask Type: Impedance Measurement model
      mask Description: Simulink model for the Impedance Measurement block. The model  injects a null current in the circuit.
  Measurement_Amplitude : ComplexToMagnitudeAngle  Output=Magnitude
  Measurement_MagnitudeAngle : Subsystem
  Measurement_RealImag : Subsystem
  SM_mechanics : Subsystem
  SSM_mechanics : Subsystem
  asynchronous_machine : Subsystem
  breaker : Subsystem  mask(Switch logic model){istate=0, Nsw=1, Rsw=1, Ts=0}
      mask prompts: Nsw "Number of switches"; Rsw "Breaker Resistances"
      mask help: Simulink model for the Ideal Switch block during a continuous simulation. The switching logic of the ideal switch is handled by the sfun_psbcontc.c function.
  distributed_param_line : Subsystem  mask(Distributed Parameter Line Model){nphase=Phases, f=Frequency, ri=Resistance, li=Inductance, ci=Capacitance, long=Length, V1_init=x1, V2_init=x2, I1_init=x3, I2_init=x4, time_init=x5}
      mask prompts: nphase "Number of phases"; f "Frequency used for R L C specification (Hz)"; ri "R [3*3 matrix] or [R0 R1] (ohms/km)"; li "L [3*3matrix ] or [L0 L1] (H/km)"; ci "C [3*3matrix] or [C0 C1] (F/km)"; long "Line length (km)"; time_init "time delay init"
      mask help: Simulink model for the Distributed Parameter Line block. The last five parameters are automatically calculated by SimPowerSystems at the begining of the simulation.
      mask init:
      | [Zm,R,v,Ti]=powericon('Distributed Parameter Line Model',nphase,f,ri,li,ci);to=long./v;Rt4=R*long/4;h=(Zm-Rt4)./(Zm+Rt4);
  ideal_switch : Subsystem  mask(Switch logic model){Nsw=1, Rsw=1, Ts=0}
      mask prompts: Nsw "Number of switches"; Rsw "Switch resistances"
      mask help: Simulink model for the Ideal Switch block during a continuous simulation. The switching logic of the ideal switch is handled by the sfun_psbcontc.c function.
  simplified_sync_mach : Subsystem
  synchronous_machine : Subsystem

== system powerlib_models/Sources ==
  ACSource : Sin  Amplitude=Amplitude  Frequency=2*pi*Frequency  Phase=Phase*pi/180  SampleTime=SampleTime
  ACSource_Cmplx : Constant  Value=complex(Amplitude*cos(Phase*pi/180),Amplitude*sin(Phase*pi/180))
  DCVoltageSource : Constant  Value=Amplitude
  DCVoltageSource_Cmplx : Constant  Value=complex(Amplitude,0)
  ThreePhaseSource : Subsystem
  ThreePhaseSource_Cmplx : Subsystem

== system powerlib_models/Switch Current Source ==
  IGBT : Subsystem  mask(IGBT model){Ron=0.01, Lon=1e-6, Vf=1, Tf=10e-6, Tt=20e-6, IC=0}
      mask prompts: Ron "Resistance Ron (Ohms) :"; Lon "Inductance Lon (H) :"; Vf "Forward voltage Vf (V) :"; Tf "Current 10% fall time Tf (s) :"; Tt "Current tail time Tt (s):"; IC "Initial current Ic (A) :"
      mask help: Simulink model for the IGBT blockt. In on-state, the IGBT model has an internal resistance (Ron) and an inductance (Lon). Lon cannot be set to zero. In off-state, the IGBT model has an infinite impedance. Discretization of the IGBTblock is available only through the Universal Bridge block.
  detailed_thyristor : Subsystem  mask(Thyristor model){Ron=1e-2, Lon=10e-6, Vf=0.8, IL=0.1, Tq=100e-6, IC=0}
      mask prompts: Ron "Resistance Ron (Ohms) :"; Lon "Inductance Lon (H) :"; Vf "Forward voltage Vf (V) :"; IL "Latching current Il (A) :"; Tq "Turn-off time Tq (s) :"; IC "Initial current Ic (A) :"
      mask help:
      | Simulates a thyristor in parallel with a series Rs-Cs snubber circuit. In on-state thyristor has internal resistance (Ron) and inductance (Lon - required by model, cannot be set to zero). In off-state thyristor impedance is infinite.
      |
      | Input one is Vak and input two is the gate signal .
      | Output one is Iak and output two is the measurement output vector [Iak Vak].
  diode : Subsystem  mask(Diode model){Ron=0.01, Lon=1e-6, Vf=0.8, IC=0}
      mask prompts: Ron "Resistance Ron (Ohms) :"; Lon "Inductance Lon (H) :"; Vf "Forward voltage Vf (V) :"; IC "Initial current Ic (A) :"
      mask help: Simulink model for the Diode block when Lon >0. In on-state, the diode has an internal resistance (Ron) and an inductance (Lon). Lon cannot be set to zero. In off-state, the diode impedance is infinite. Input one is Vak. Output one is Iak and output 2 is the measurement output vector [Iak Vak].
  gto : Subsystem  mask(Gto model){Ron=0.001, Lon=1e-5, Vf=0.8, Tf=200e-6, Tt=200e-6, IC=0}
      mask prompts: Ron "Resistance Ron (Ohms) :"; Lon "Inductance Lon (H) :"; Vf "Forward voltage Vf (V) :"; Tf "Current 10% fall time Tf (s) :"; Tt "Current tail time Tt (s) :"; IC "Initial current Ic (A) :"
      mask help: Simulink model for the GTO block. In on-state, the GTO has an internal resistance (Ron) and an inductance (Lon). Lon cannot be set to zero. In off-state, the GTO impedance is infinite. Input one is Vak and input two is the Gate signal. Output one is Iak and output 2 is the measurement output vector [Iak Vak].
  mosfet : Subsystem  mask(Mosfet model ){Ron=0.001, Lon=0.05, Rd=1e-6, IC=0}
      mask prompts: Ron "MOSFET resistance Ron (Ohms) :"; Lon "MOSFET inductance Lon (H) :"; Rd "Internal diode resistance Rd (Ohms) :"; IC "Initial current Ic (A) :"
      mask help: Simulink model for the MOSFETblock. the model simulate an internal diode in parallel with the MOSFET. In on-state, the MOSFET has an internal resistance (Ron if Ids>0 , Rd if Ids<0) and an inductance (Lon). Lon cannot be set to zero). In off-state, the MOSFET impedance is infinite. Input one is Vds and input two is the Gate signal. Output one is Ids and output 2 is the measurement output vector [Ids Vds].
      mask init:
      | ICmos=abs(IC).*(IC>0);
      | ICdiode=abs(IC).*(IC<0);
  thyristor : Subsystem  AncestorBlock=powerlib_models/Switch Current Source/thyristor_GS  mask(Thyristor s model){Ron=1, Lon=10e-6, Vf=0.8, IC=47e-6}
      mask prompts: Ron "Resistance Ron (Ohms) :"; Lon "Inductance Lon (H) :"; Vf "Forward voltage Vf (V) :"; IC "Initial current Ic (A) :"
      mask help: Simulink model for the Thyristor block when Lon>0. In on-state, the thyristor has an internal resistance (Ron) and an inductance (Lon). Lon cannot be set to zero. In off-state, the thyristor impedance is infinite. Input one is Vak and input two is the gate signal. Output one is Iak and output two is the measurement output vector [Iak Vak].
